simulink library "tqd"  (R2021b)
settings: Solver=VariableStepAuto  StartTime=0.0  StopTime=10.0  RelTol=1e-3
undefined symbols (not defined in the file or in its folder): ATQD_APSDecReq_X_kph, ATQD_APSDecReq_Y_mps2, ATQD_APSDecReqCMD_X_kph, ATQD_APSDecReqTs_X_pct, ATQD_APSDecTimeGain_X_Deg, ATQD_APSDecTimeGain_Y_s, ATQD_APSReqLowSpd_X_Deg, ATQD_AutoHoldReleaseBPS_X_Deg, ATQD_AWDLoadTrqnsGain_X_kg, ATQD_AWDLoadTrqnsGain_Y_pct, ATQD_BOSEnBPSPosn_X_kph, ATQD_BOSMap_X_rpm, ATQD_BOSMap_Y_pct, ATQD_CreepBaseTqD_X_kph, ATQD_CreepBaseTqD_Y_Deg, ATQD_CreepBaseTqR_X_kph, ATQD_CreepBaseTqR_Y_Deg, ATQD_CreepBPSDisPosn_X_Deg, ATQD_CreepBPSDisPosnR_X_Deg, ATQD_CreepBPSEnPosn_X_Deg, ATQD_CreepBPSEnPosnR_X_Deg, ATQD_CreepDeltaTq_X_kph, ATQD_CreepIterm_X_kph, ATQD_CreepIterm_Y_kph, ATQD_CreepItermMaxLimit_X_pct, ATQD_CreepPreloadTime_X_kph, ATQD_CreepPreloadTq_X_kph, ATQD_CreepPreloadTq_Y_s, ATQD_CreepProtTq_X_Deg, ATQD_CreepPterm_X_kph, ATQD_ECOTqMapD_X_rpm, ATQD_ECOTqMapD_Y_pct, ATQD_EOPDTqMapDCon_X_rpm, ATQD_EOPDTqMapDCon_Y_Deg, ATQD_EstInitVehWeight_X_c, ATQD_LHMRollGenMapD_X_rpm, ATQD_LHMRollGenMapD_Y_rpm, ATQD_LHMTqMapD_X_rpm, ATQD_LHMTqMapD_Y_pct, ATQD_NL1TqMapD_X_rpm, ATQD_NL1TqMapD_Y_pct, ATQD_NOPDTqMapDCon_X_rpm, ATQD_NOPDTqMapDCon_Y_Deg, ATQD_NRMRrEDUSpRat_X_rpm, ATQD_NRMRrEDUSpRat_Y_Nm, ATQD_OPDHoldDownRelDelay_X_Deg, ATQD_OPDHoldEnSpd_X_Deg, ATQD_OPDHoldRelDetTime_X_Deg, ATQD_OPDHoldReleaseTq_X_Deg, ATQD_OrigPedTqLowLim_X_Deg, ATQD_OrigPedTqLowLim_Y_pct, ATQD_PedalMapClimbUpLim_X_rpm, ATQD_PedalMapClimbUpLim_Y_Deg, ATQD_PreLoadTq_X_s, ATQD_RollGenMapEL1_X_rpm, ATQD_RollGenMapEL1_Y_rpm, ATQD_SL1TqMapD_X_rpm, ATQD_SL1TqMapD_Y_pct, ATQD_SlideRegenTqGain_X_Gps, ATQD_SlideRegenTqGain_Y_pct ... (+378)
libraries: hcu_lib x59, simulink x49
(part 12 of 12)

== system tqd/TQD/TorqueDemand/TorqueModule/DriverWhlTqDem/PedalMapWhlTq/NoLHM/ShiftD/LUT_D_Sport/Sport_Lv5_TqMap ==
  VTQD_SL5TqMapDIn_Nm : Inport
  Action Port : ActionPort
  VTQD_SL5TqMapDOut_Nm : Outport
  wires:
  VTQD_SL5TqMapDIn_Nm/1 -> VTQD_SL5TqMapDOut_Nm/1

== system tqd/TQD/TorqueDemand/TorqueModule/DriverWhlTqDem/PedalMapWhlTq/NoLHM/ShiftD/LUT_D_Sport/Sport_OnePedal_TqMap ==
  VTQD_SOPDTqMapDIn_Nm : Inport
  VTQD_SOPDTqMapDCon_Nm : Inport  Port=2
  VTQD_APSReqTimer_s : Inport  Port=3
  VTQD_LowIdleAccPedal_flg : Inport  Port=4
  VTQD_OPDHoldEnRel_flg : Inport  Port=5
  VTQD_OPDHoldActRelTq_Nm : Inport  Port=6
  VTQD_VehActSpd_kph : Inport  Port=7
  VTQD_SlopeUp_flg : Inport  Port=8
  Action Port : ActionPort
  AND : Logic  AllPortsSameDT=off  OutDataTypeStr=boolean
  Add : Sum
  Constant1 : Constant  Value=ZERO_FLOAT
  Constant2 : Constant  Value=KTQD_OPDHTqDisComSpd_kph
  Constant9 : Constant  Value=KTQD_APSReqDelayTime_s
  Detect Increase : simulink/Logic and Bit Operations/Detect Increase  vinit=0.0  OutDataTypeStr=boolean
  Max : MinMax  Function=max  Inputs=2
  NOT : Logic  Operator=NOT  AllPortsSameDT=off  OutDataTypeStr=boolean
  OR : Logic  Operator=OR  Inputs=3  AllPortsSameDT=off  OutDataTypeStr=boolean
  Relational Operator : RelationalOperator  Operator=>  OutDataTypeStr=boolean  RndMeth=Simplest
  Relational Operator2 : RelationalOperator  OutDataTypeStr=boolean  RndMeth=Simplest
  SR_Latch : hcu_lib/Basic_Blocks/SR_Latch
  Switch : Switch  Criteria=u2 > Threshold
  Switch1 : Switch  Criteria=u2 > Threshold
  VTQD_SOPDTqMapDOut_Nm : Outport
  wires:
  Constant1/1 -> Switch/1
  VTQD_SOPDTqMapDCon_Nm/1 -> Switch/3
  VTQD_APSReqTimer_s/1 -> Relational Operator2/1
  Switch/1 -> Add/2
  Constant9/1 -> Relational Operator2/2
  VTQD_SOPDTqMapDIn_Nm/1 -> Add/1
  AND/1 -> Switch/2
  Relational Operator2/1 -> AND/1
  Switch1/1 -> VTQD_SOPDTqMapDOut_Nm/1
  VTQD_LowIdleAccPedal_flg/1 -> [VTQD_LowIdleAccPedal_flg]
  [VTQD_LowIdleAccPedal_flg] -> AND/2
  NOT/1 -> OR/3
  Relational Operator/1 -> OR/2
  VTQD_OPDHoldActRelTq_Nm/1 -> Max/2
  [VTQD_LowIdleAccPedal_flg] -> OR/1
  Max/1 -> Switch1/1
  VTQD_OPDHoldEnRel_flg/1 -> Detect Increase/1
  VTQD_VehActSpd_kph/1 -> Relational Operator/1
  Detect Increase/1 -> SR_Latch/1
  Add/1 -> Max/1, Switch1/3
  OR/1 -> SR_Latch/2
  SR_Latch/1 -> Switch1/2
  Constant2/1 -> Relational Operator/2
  VTQD_SlopeUp_flg/1 -> NOT/1

== stateflow chart tqd/TQD/TorqueDemand/Signal_convert/Chart ==
  state Creep_function_switch
    (default) -> (junction 12) : { VTQD_SaveCreepSW_flg =FALSE;}
    Creep_function_switch -> (junction 12)
    (junction 12) -> (junction 16) [order 1] : [VPMM_SysPowerMode_enum != ENUM_PWRSTASW_STANDBY ]
    (junction 12) -> (junction 19) [order 2] : {VTQD_CreepON_flg = TRUE;
        |  VTQD_SaveCreepSW_flg = VTQD_CreepON_flg;}
    (junction 16) -> (junction 23)
    (junction 23) -> (junction 25) [order 1] : [KTQD_CreepSW_flg_ovrdflg != TRUE]
    (junction 23) -> (junction 28) [order 2] : {VTQD_CreepON_flg = KTQD_CreepSW_flg_ovrdval;}
    (junction 25) -> (junction 30)
    (junction 30) -> (junction 32) [order 1] : [VINP_RegenMode_enum != ENUM_REGENLEVEL_OPD]
    (junction 30) -> (junction 34) [order 2] : {VTQD_CreepON_flg = FALSE;}
    (junction 32) -> (junction 37)
    (junction 37) -> (junction 39) [order 1] : [VTQD_OPDOn2Off_flg != TRUE]
    (junction 37) -> (junction 42) [order 2] : {VTQD_CreepON_flg = VTQD_SaveCreepSW_flg;}
    (junction 39) -> (junction 45)
    (junction 45) -> (junction 47) [order 1] : [VINP_IVICreepSWReq_flg == TRUE]
    (junction 45) -> (junction 49) [order 2] : {VTQD_CreepON_flg = VTQD_LastCreepON_flg;}
    (junction 47) -> (junction 51)
    (junction 51) -> (junction 53) [order 1] : [VTQD_LastCreepON_flg != FALSE]
    (junction 51) -> (junction 55) [order 2] : {VTQD_CreepON_flg = TRUE;
        |  VTQD_SaveCreepSW_flg = VTQD_CreepON_flg;}
    (junction 53) -> (junction 57) : {VTQD_CreepON_flg = FALSE;
        |  VTQD_SaveCreepSW_flg = VTQD_CreepON_flg;}
  (default) -> Creep_function_switch
  data: VPMM_SysPowerMode_enum input; KTQD_CreepSW_flg_ovrdflg input; KTQD_CreepSW_flg_ovrdval input; VTQD_OPDOn2Off_flg input; VINP_RegenMode_enum input; VTQD_LastCreepON_flg input; VINP_IVICreepSWReq_flg input; ENUM_PWRSTASW_STANDBY parameter; TRUE parameter; VTQD_CreepON_flg output boolean; ENUM_REGENLEVEL_OPD parameter; FALSE parameter; VTQD_SaveCreepSW_flg local boolean

== stateflow chart tqd/TQD/TorqueDemand/ShiftModule/Determine_Actual_Gear_Position ==
  state Initialize [commented out]
    en:
    VTQD_GearActualPosn_enum = ENUM_GEARACTUALPOSN_INVALID;
    VTQD_ShiftInitialComplete_flg = FALSE;
    (default) -> (junction 489) [commented out] : {
        | VTQD_InitializeTime_s = 0;
        | }
    Initialize -> (junction 489) [commented out]
    (junction 489) -> (junction 490) [commented out] : [VTQD_InitializeTime_s > KTQD_ShiftInitialTime_s]
    (junction 489) -> (junction 531) [commented out] : {
        | VTQD_InitializeTime_s = VTQD_InitializeTime_s + task_time_s;
        | }
    (junction 490) -> (junction 533) [commented out] : {
        | VTQD_ShiftInitialComplete_flg = TRUE;
        | }
    (junction 533) -> (junction 531) [commented out]
  state PBW_Judgement [commented out]
    en:
    VTQD_PBWReleased_flg = FALSE;
    VTQD_PBWLocked_flg = FALSE;
    VTQD_PBWUnlockTO_flg = FALSE;
    VTQD_PBWLockTO_flg = FALSE;
    state Initialize [commented out]
      en:
      VTQD_PBWUnlockTO_flg = FALSE;
      VTQD_PBWReleased_flg = FALSE;
      VTQD_PBWLocked_flg = FALSE;
    state PBWUnlock [commented out]
      en:
      VTQD_ParkRequest_flg = FALSE;
      (default) -> (junction 798) [commented out] : {
          | VTQD_PBWWaitTime_s = 0;
          | }
      PBWUnlock -> (junction 798) [commented out]
      (junction 798) -> (junction 799) [commented out] : [VINP_PBWMotorPos_enum == ENUM_PBWPOSITION_UNPARKED]
      (junction 798) -> (junction 800) [commented out] : {
          | VTQD_PBWWaitTime_s += task_time_s;
          | }
      (junction 799) -> (junction 804) [commented out] : {
          | VTQD_PBWReleased_flg = TRUE;
          | }
      (junction 800) -> (junction 801) [commented out] : [VTQD_PBWWaitTime_s >= KTQD_PBWTimeout_s]
      (junction 800) -> (junction 802) [commented out]
      (junction 801) -> (junction 803) [commented out] : {
          | VTQD_PBWUnlockTO_flg = TRUE;
          | }
      (junction 803) -> (junction 802) [commented out]
      (junction 804) -> (junction 803) [commented out]
    state PBWLock [commented out]
      en:
      VTQD_ParkRequest_flg = TRUE;
      (default) -> (junction 817) [commented out] : {
          | VTQD_PBWWaitTime_s = 0;
          | }
      (junction 817) -> (junction 816) [commented out] : [VINP_PBWMotorPos_enum == ENUM_PBWPOSITION_PARKED]
      PBWLock -> (junction 817) [commented out]
      (junction 816) -> (junction 822) [commented out] : {
          | VTQD_PBWLocked_flg = TRUE;
          | }
      (junction 817) -> (junction 818) [commented out] : {
          | VTQD_PBWWaitTime_s += task_time_s;
          | }
      (junction 818) -> (junction 819) [commented out] : [VTQD_PBWWaitTime_s >= KTQD_PBWTimeout_s]
      (junction 818) -> (junction 820) [commented out]
      (junction 819) -> (junction 821) [commented out] : {
          | VTQD_PBWLockTO_flg = TRUE;
          | }
      (junction 821) -> (junction 820) [commented out]
      (junction 822) -> (junction 821) [commented out]
    (default) -> PBW_Judgement.Initialize [commented out]
    PBW_Judgement.Initialize -> PBWUnlock [commented out] : [VTQD_GearShiftCMD_enum != ENUM_GEARSHIFTCMD_P]
    PBW_Judgement.Initialize -> PBWLock [commented out] : [VTQD_GearShiftCMD_enum == ENUM_GEARSHIFTCMD_P]
  state N
    en:
    VTQD_GearActualPosn_enum = ENUM_GEARACTUALPOSN_N;
    VTQD_ParkRequest_flg = FALSE;
    VTQD_EnterP_flg = FALSE;
    (default) -> (junction 753) : {
        | VTQD_RelockWaitTime_s = 0;
        | }
    (junction 753) -> (junction 754) [order 1] : %[!VTQD_PBWLockTO_flg]
    N -> (junction 753) [order 1]
    (junction 753) -> (junction 755) [order 2] : {
        | VTQD_RelockWaitTime_s += task_time_s;
        | }
    (junction 754) -> (junction 757) : {
        | VTQD_EnterP_flg = TRUE;
        | }
    (junction 755) -> (junction 756) [order 1] : [VTQD_RelockWaitTime_s >= KTQD_RelockWaitTime_s]
    (junction 755) -> (junction 760) [order 2]
    (junction 756) -> (junction 758) : {
        | VTQD_EnterP_flg = TRUE;
        | }
    (junction 758) -> (junction 760)
    (junction 757) -> (junction 758)
  state P
    en:
    VTQD_GearActualPosn_enum = ENUM_GEARACTUALPOSN_P;
    VTQD_ParkRequest_flg = TRUE;
    VTQD_ExitP_flg = FALSE;
    (default) -> (junction 636) : {
        | VTQD_ReunlockWaitTime_s = 0;
        | }
    P -> (junction 636) [order 1]
    (junction 636) -> (junction 641) [order 1] : %[!VTQD_PBWUnlockTO_flg]
    (junction 636) -> (junction 645) [order 2] : {
        | VTQD_ReunlockWaitTime_s += task_time_s;
        | }
    (junction 641) -> (junction 637) : {
        | VTQD_ExitP_flg = TRUE;
        | }
    (junction 645) -> (junction 632) [order 1] : [VTQD_ReunlockWaitTime_s >= KTQD_ReunlockWaitTime_s]
    (junction 645) -> (junction 647) [order 2]
    (junction 632) -> (junction 643) : {
        | VTQD_ExitP_flg = TRUE;
        | }
    (junction 643) -> (junction 647)
    (junction 637) -> (junction 643)
  state D
    en:
    VTQD_GearActualPosn_enum = ENUM_GEARACTUALPOSN_D;
    VTQD_ParkRequest_flg = FALSE;
  state R
    en:
    VTQD_GearActualPosn_enum = ENUM_GEARACTUALPOSN_R;
    VTQD_ParkRequest_flg = FALSE;
  (default) -> P : {
      |  VTQD_PBWLockTO_flg = FALSE;
      |  VTQD_PBWUnlockTO_flg = FALSE;
      | }
  N -> (junction 731) [order 2] : [VTQD_GearShiftCMD_enum == ENUM_GEARSHIFTCMD_R && VTQD_PwrStaAllowDR_flg &&...
      |  VTQD_TMRotateDirction_enum ~= ENUM_TMROTATEDIRECTACT_FORWARD &&...
      | (VTQD_BrkSwSta_flg || VVMC_APSActive_flg) && !VINP_EPBCarWashMode_flg]
  P -> N [order 1] : [(VTQD_GearShiftCMD_enum == ENUM_GEARSHIFTCMD_N &&...
      | VTQD_PwrStaAllowPN_flg && (VTQD_BrkSwSta_flg || VVMC_APSActive_flg) && VTQD_ExitP_flg)&&...
      | !VTQD_ForceP_flg]
      | %add20240308
  (junction 731) -> (junction 733)
  (junction 749) -> N
  N -> P [order 3] : [(VTQD_GearShiftCMD_enum == ENUM_GEARSHIFTCMD_P && VTQD_PwrStaAllowPN_flg &&...
      |  VINP_VehSpd_kph <= KTQD_VehSpd2P_kph && VTQD_EnterP_flg) || VTQD_ForceP_flg ]
      | %add20240308
  (junction 747) -> (junction 749)
  D -> N [order 1] : [VTQD_GearShiftCMD_enum == ENUM_GEARSHIFTCMD_N ||...
      | !VTQD_PwrStaAllowDR_flg ||...
      | VINP_EPBCarWashMode_flg]
  N -> D [order 1] : [VTQD_GearShiftCMD_enum == ENUM_GEARSHIFTCMD_D && VTQD_PwrStaAllowDR_flg &&...
      |  VTQD_TMRotateDirction_enum ~= ENUM_TMROTATEDIRECTACT_REVERSE &&...
      | !VINP_EPBCarWashMode_flg]
  P -> D [order 2] : [VTQD_GearShiftCMD_enum == ENUM_GEARSHIFTCMD_D &&...
      | VTQD_PwrStaAllowDR_flg && (VTQD_BrkSwSta_flg || VVMC_APSActive_flg) && VTQD_ExitP_flg &&...
      |  !VTQD_ForceP_flg]
      | %add20240308
  D -> P [order 2] : [(VTQD_GearShiftCMD_enum == ENUM_GEARSHIFTCMD_P && VTQD_PwrStaAllowPN_flg &&...
      |  VINP_VehSpd_kph <= KTQD_VehSpd2P_kph) || VTQD_ForceP_flg]
      | %add20240308
  R -> D [order 3] : [VTQD_GearShiftCMD_enum == ENUM_GEARSHIFTCMD_D && VTQD_PwrStaAllowDR_flg &&...
      | ( VTQD_BrkSwSta_flg ||VVMC_APSActive_flg) &&...
      | VINP_VehSpd_kph <= KTQD_VehSpdRev_kph]
  D -> R [order 3] : [VTQD_GearShiftCMD_enum == ENUM_GEARSHIFTCMD_R && VTQD_PwrStaAllowDR_flg &&...
      |  (VTQD_BrkSwSta_flg || VVMC_APSActive_flg) &&...
      | VINP_VehSpd_kph <= KTQD_VehSpdRev_kph]
  P -> R [order 3] : [VTQD_GearShiftCMD_enum == ENUM_GEARSHIFTCMD_R &&...
      | VTQD_PwrStaAllowDR_flg && (VTQD_BrkSwSta_flg || VVMC_APSActive_flg) && VTQD_ExitP_flg && !VTQD_ForceP_flg]
      | %add20240308
  R -> (junction 747) [order 1] : [VTQD_GearShiftCMD_enum == ENUM_GEARSHIFTCMD_N ||...
      | !VTQD_PwrStaAllowDR_flg ||...
      | VINP_EPBCarWashMode_flg]
  (junction 733) -> R
  R -> P [order 2] : [(VTQD_GearShiftCMD_enum == ENUM_GEARSHIFTCMD_P && VTQD_PwrStaAllowPN_flg &&...
      |  VINP_VehSpd_kph <= KTQD_VehSpd2P_kph) || VTQD_ForceP_flg]
      | %add20240308
  data: task_time_s input; VTQD_BrkSwSta_flg input; VTQD_GearShiftCMD_enum input; VINP_VehSpd_kph input; VINP_PBWMotorPos_enum input; VTQD_PwrStaAllowDR_flg input; VTQD_PwrStaAllowPN_flg input; VTQD_TMRotateDirction_enum input; VTQD_GearActualPosn_enum output uint8; ENUM_GEARACTUALPOSN_N parameter; ENUM_GEARACTUALPOSN_D parameter; ENUM_GEARACTUALPOSN_R parameter; ENUM_GEARACTUALPOSN_P parameter; KTQD_VehSpd2P_kph input; VTQD_InitializeTime_s local single; ENUM_GEARACTUALPOSN_INVALID parameter; FALSE parameter; TRUE parameter; VTQD_ShiftInitialComplete_flg local boolean; ENUM_GEARSHIFTCMD_D parameter; ENUM_GEARSHIFTCMD_P parameter; ENUM_GEARSHIFTCMD_R parameter; ENUM_GEARSHIFTCMD_N parameter; KTQD_VehSpdRev_kph input; KTQD_ShiftInitialTime_s input; ENUM_PBWPOSITION_PARKED parameter; ENUM_PBWPOSITION_UNPARKED parameter; VTQD_PBWLockTO_flg output boolean; VTQD_PBWUnlockTO_flg output boolean; KTQD_PBWTimeout_s input; KTQD_RelockWaitTime_s input; KTQD_ReunlockWaitTime_s input; VTQD_ParkRequest_flg output boolean; VTQD_EnterP_flg local boolean; VTQD_ExitP_flg local boolean; VTQD_PBWLocked_flg local boolean; VTQD_PBWReleased_flg local boolean; VTQD_PBWWaitTime_s local single; VTQD_RelockWaitTime_s local single; VTQD_ReunlockWaitTime_s local single; ENUM_TMROTATEDIRECTACT_FORWARD parameter; ENUM_TMROTATEDIRECTACT_REVERSE parameter; VINP_EPBCarWashMode_flg input; VVMC_APSActive_flg input; VTQD_ForceP_flg input
